simulink model "VendingMachine"  (R2020a)
settings: Solver=VariableStepAuto  StartTime=0.0  StopTime=1000  RelTol=1e-3
settings Model: EnablePacing=on  PacingRate=10  Creator=vivek vivian  LastModifiedBy=vivek vivian

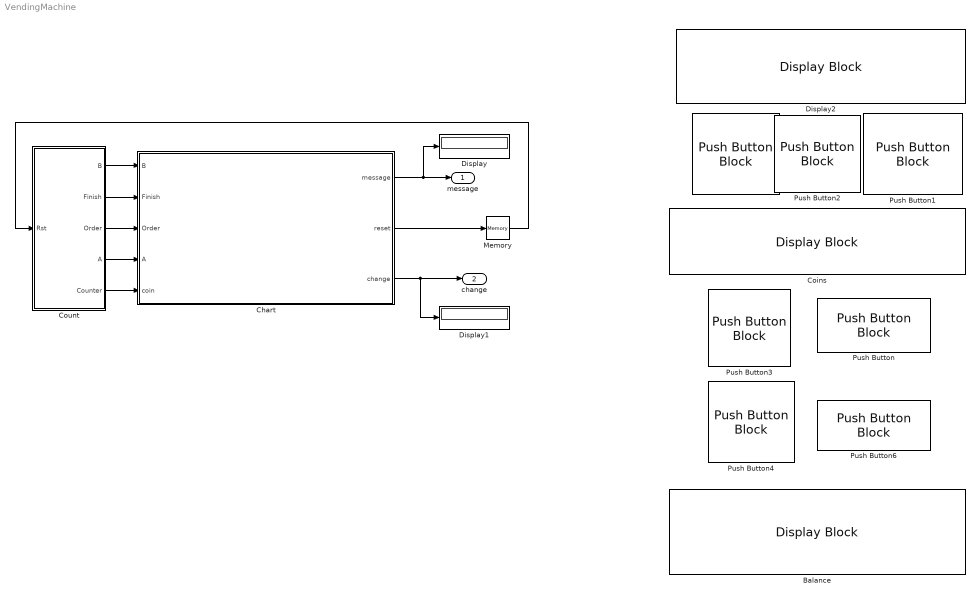
== system VendingMachine ==
  " " : PushButtonBlock  ButtonText=1kr
  Balance : DisplayBlock  LabelPosition=Hide  Format=short  Transparency=1
  Chart : Stateflow chart  TreatAsAtomicUnit=on
  Coins : DisplayBlock  LabelPosition=Hide  Format=short  Transparency=1
  Count : Subsystem
  Display : Display
  Display1 : Display
  Display2 : DisplayBlock  LabelPosition=Hide  Format=short  Transparency=1
  Memory : Memory
  Push Button : PushButtonBlock  ButtonText=Order
  Push Button1 : PushButtonBlock  ButtonText=10kr  OnValue=10
  Push Button2 : PushButtonBlock  ButtonText=5kr  OnValue=5
  Push Button3 : PushButtonBlock  ButtonText=A  OnValue=100
  Push Button4 : PushButtonBlock  ButtonText=B  OnValue=100
  Push Button6 : PushButtonBlock  ButtonText=Finish
  message : Outport
  change : Outport  Port=2
  wires:
  Count/5(Counter) -> Chart/5(coin)
  Count/4(A) -> Chart/4(A)
  Count/3(Order) -> Chart/3(Order)
  Count/2(Finish) -> Chart/2(Finish)
  Count/1(B) -> Chart/1(B)
  Chart/1(message) -> Display/1, message/1
  Chart/3(change) -> Display1/1, change/1
  Chart/2(reset) -> Memory/1
  Memory/1 -> Count/1(Rst)

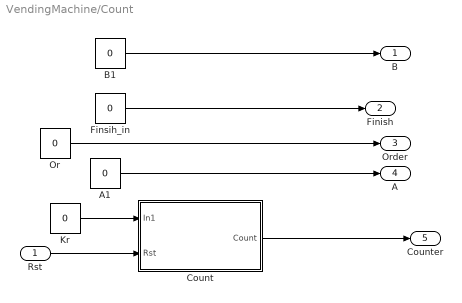
== system VendingMachine/Count ==
  Rst : Inport
  A1 : Constant  Value=0
  B1 : Constant  Value=0
  Count : Subsystem
  Finsih_in : Constant  Value=0
  Kr : Constant  Value=0  OutDataTypeStr=double
  Or : Constant  Value=0
  B : Outport
  Finish : Outport  Port=2
  Order : Outport  Port=3
  A : Outport  Port=4
  Counter : Outport  Port=5
  wires:
  Or/1 -> Order/1
  Kr/1 -> Count/1(In1)
  A1/1 -> A/1
  B1/1 -> B/1
  Count/1(Count) -> Counter/1
  Finsih_in/1 -> Finish/1
  Rst/1 -> Count/2(Rst)

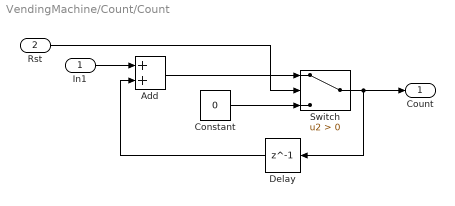
== system VendingMachine/Count/Count ==
  In1 : Inport
  Rst : Inport  Port=2
  Add : Sum
  Constant : Constant  Value=0
  Delay : Delay  DelayLength=1
  Switch : Switch  Criteria=u2 > Threshold
  Count : Outport
  wires:
  Add/1 -> Switch/1
  In1/1 -> Add/1
  Constant/1 -> Switch/3
  Switch/1 -> Delay/1, Count/1
  Rst/1 -> Switch/2
  Delay/1 -> Add/2

== stateflow chart VendingMachine/Chart ==
  state Order_State
    message = "Enter A or B";
  state Inserting_State
    message = "Insert Coins!";
    du:coins=coin;
    ex:change=change+coins;
  state Idle_State
    en:coins=0;reset=1;change=0;
    du:coins=coin;
    message="Welcome";
  state Product_A
    en:reset=0;change=change-8;
    ex:reset=1;
  state Return_Change
    message="Collect Change!"
  state Prdocut_B
    en:reset=0;change=change-6;
    ex:reset=1;
  state Insufficient_Balance
    message="Sorry Try Again";
  state Order_More_Snacks
  state Finish
    message="Thank You!";
    reset=0
  Return_Change -> Idle_State
  Inserting_State -> Order_State : [Order>0]
  Order_State -> Inserting_State [order 3] : [change<=6&&B>0||A>0]
  Order_More_Snacks -> Order_State [order 2]
  Idle_State -> Inserting_State : [coins>1]
  (default) -> Idle_State
  Order_State -> Prdocut_B [order 2] : [B>0&&change>=6]
  Order_State -> Product_A [order 1] : [A>0&&change>=8]
  Order_More_Snacks -> Inserting_State [order 1] : [coins<=8]{coins=0}
  Insufficient_Balance -> Inserting_State
  Product_A -> Order_More_Snacks [order 2] : [Order==1]{coins=change}
  Product_A -> Finish [order 3] : [Finish==1]
  Product_A -> Insufficient_Balance [order 1] : [change<8&&Order==1]
  Prdocut_B -> Order_More_Snacks [order 3] : [Order==1]{coins=change}
  Prdocut_B -> Finish [order 2] : [Finish==1]
  Prdocut_B -> Insufficient_Balance [order 1] : [change<6&&Order==1]
  Finish -> Idle_State [order 2]
  Finish -> Return_Change [order 1] : [change>0]
  data: B input; Finish input; Order input; A input; coin input; message output string; reset output; change output; coins local double
